simulink library "AerodynamicModel"  (R2024a)
settings: Solver=ode45  StartTime=0.0  StopTime=10.0  RelTol=1e-3  EnableMultiTasking=on
values from neighbouring files (symbols this model uses):
  b = 5.76    [Initialization.m]    (also in Initialization_alt2.m; Initialization_cg1.m; Initialization_loop.m; Initialization_v2.m)
  CD0 = 0.01534    [Initialization.m]    (also in Initialization_alt2.m; Initialization_cg1.m = 0.01532; Initialization_loop.m = 0.01533; Initialization_v2.m)
  CD_alpha = 0    [Initialization.m]    (also in Initialization_alt2.m; Initialization_cg1.m; Initialization_loop.m; Initialization_v2.m)
  CD_elev = 0.000010*180/pi    (= 0.000572957795131)    [Initialization.m]    (also in Initialization_alt2.m; Initialization_cg1.m; Initialization_loop.m; Initialization_v2.m)
  CL0 = 0.20539    [Initialization.m]    (also in Initialization_alt2.m; Initialization_cg1.m; Initialization_loop.m; Initialization_v2.m)
  Cl_ail = 0.005020*180/pi    (= 0.287624813156)    [Initialization.m]    (also in Initialization_alt2.m; Initialization_cg1.m; Initialization_loop.m = 0.276051065694; Initialization_v2.m)
  CL_alpha = 4.865906    [Initialization.m]    (also in Initialization_alt2.m = 4.865879; Initialization_cg1.m; Initialization_loop.m = 4.86588; Initialization_v2.m = 4.865879)
  CL_AlphaDot = 0    [Initialization.m]    (also in Initialization_alt2.m; Initialization_cg1.m; Initialization_loop.m; Initialization_v2.m)
  Cl_beta = -0.020876    [Initialization.m]    (also in Initialization_alt2.m; Initialization_cg1.m; Initialization_loop.m; Initialization_v2.m)
  CL_elev = 0.0064*180/pi    (= 0.366692988884)    [Initialization.m]    (also in Initialization_alt2.m; Initialization_cg1.m; Initialization_loop.m; Initialization_v2.m)
  Cl_p = -0.464911    [Initialization.m]    (also in Initialization_alt2.m; Initialization_cg1.m = -0.464912; Initialization_loop.m; Initialization_v2.m = -0.464912)
  CL_q = 8.057645    [Initialization.m]    (also in Initialization_alt2.m = 7.535819; Initialization_cg1.m = 7.53583; Initialization_loop.m = 8.688618; Initialization_v2.m = 7.535819)
  Cl_r = 0.073227    [Initialization.m]    (also in Initialization_alt2.m = 0.072902; Initialization_cg1.m = 0.099393; Initialization_loop.m = 0.073622; Initialization_v2.m = 0.099393)
  Cl_rud = -0.000235*180/pi    (= -0.0134645081856)    [Initialization.m]    (also in Initialization_alt2.m; Initialization_cg1.m; Initialization_loop.m; Initialization_v2.m)
  Cm0 = -0.05304    [Initialization.m]    (also in Initialization_alt2.m = -0.04206; Initialization_cg1.m = -0.04206; Initialization_loop.m = -0.06631; Initialization_v2.m = -0.04206)
  Cm_alpha = -0.985144    [Initialization.m]    (also in Initialization_alt2.m = -0.724231; Initialization_cg1.m = -0.724233; Initialization_loop.m = -1.300632; Initialization_v2.m = -0.724231)
  Cm_AlphaDot = 0    [Initialization.m]    (also in Initialization_alt2.m; Initialization_cg1.m; Initialization_loop.m; Initialization_v2.m)
  Cm_elev = -0.016898 *180/pi    (= -0.968184082212)    [Initialization.m]    (also in Initialization_alt2.m = -0.948588925619; Initialization_cg1.m = -0.948588925619; Initialization_loop.m = -0.991847239151; Initialization_v2.m = -0.948588925619)
  Cm_q = -9.625909    [Initialization.m]    (also in Initialization_alt2.m = -9.117785; Initialization_cg1.m = -9.117792; Initialization_loop.m = -10.314818; Initialization_v2.m = -9.117785)
  cma = 0.84    [Initialization.m]    (also in Initialization_alt2.m; Initialization_cg1.m; Initialization_loop.m; Initialization_v2.m)
  Cn_ail = 0.000017*180/pi    (= 0.000974028251722)    [Initialization.m]    (also in Initialization_alt2.m = 0.000859436692696; Initialization_cg1.m = 0.000916732472209; Initialization_loop.m = 0.000630253574644; Initialization_v2.m = 0.000859436692696)
  Cn_beta = 0.075240    (= 0.07524)    [Initialization.m]    (also in Initialization_alt2.m = 0.073751; Initialization_cg1.m = 0.073751; Initialization_loop.m = 0.07704; Initialization_v2.m = 0.073751)
  Cn_p = -0.012611    [Initialization.m]    (also in Initialization_alt2.m = -0.012431; Initialization_cg1.m = -0.012466; Initialization_loop.m = -0.012825; Initialization_v2.m = -0.012431)
  Cn_r = -0.076155    [Initialization.m]    (also in Initialization_alt2.m = -0.07368; Initialization_cg1.m = -0.073674; Initialization_loop.m = -0.079209; Initialization_v2.m = -0.07368)
  Cn_rud = 0.001227*180/pi    (= 0.0703019214626)    [Initialization.m]    (also in Initialization_alt2.m = 0.0690414143133; Initialization_cg1.m = 0.0690414143133; Initialization_loop.m = 0.0717916117299; Initialization_v2.m = 0.0690414143133)
  CY_ail = -0.000195*180/pi    (= -0.0111726770051)    [Initialization.m]    (also in Initialization_alt2.m; Initialization_cg1.m; Initialization_loop.m = -0.010828902328; Initialization_v2.m)
  CY_beta = -0.191039    [Initialization.m]    (also in Initialization_alt2.m; Initialization_cg1.m; Initialization_loop.m; Initialization_v2.m)
  CY_p = 0.023084    [Initialization.m]    (also in Initialization_alt2.m; Initialization_cg1.m = 0.023086; Initialization_loop.m; Initialization_v2.m)
  CY_r = 0.170019    [Initialization.m]    (also in Initialization_alt2.m = 0.167041; Initialization_cg1.m = 0.167041; Initialization_loop.m = 0.173621; Initialization_v2.m = 0.167041)
  CY_rud = -0.002799*180/pi    (= -0.160370886857)    [Initialization.m]    (also in Initialization_alt2.m; Initialization_cg1.m; Initialization_loop.m; Initialization_v2.m)
  S = 4.74    [Initialization.m]    (also in Initialization_alt2.m; Initialization_cg1.m; Initialization_loop.m; Initialization_v2.m)
settings Model: Creator=bruno  LastModifiedBy=Marcos Ramalho
settings SolverCC: AlgebraicLoopSolver=TrustRegion
settings DataIOCC: LimitDataPoints=on  ReturnWorkspaceOutputs=off
settings OptimizationCC: LifeSpan=inf
settings DebuggingCC: UnconnectedInputMsg=warning  UnconnectedOutputMsg=warning  UnconnectedLineMsg=warning  AllowSymbolicDim=off  SFUnexpectedBacktrackingDiag=warning  SFNoUnconditionalDefaultTransitionDiag=warning  ArithmeticOperatorsInVariantConditions=warning
settings ModelReferenceCC: EnableRefExpFcnMdlSchedulingChecks=on
settings SFSimCC: SimUseLocalCustomCode=off  CustomCodeUndefinedFunction=UseInterfaceOnly
settings RTWCC: RTWUseLocalCustomCode=off  GPUComputeCapability=3.5
settings CodeAppCC: StateflowObjectComments=on
settings GRTTargetCC: TargetLangStandard=C89/C90 (ANSI)
settings ConfigComp: CovMetricSettings=dw  CovSaveCumulativeToWorkspaceVar=on  CovSaveSingleToWorkspaceVar=on  CovExternalEMLEnable=off

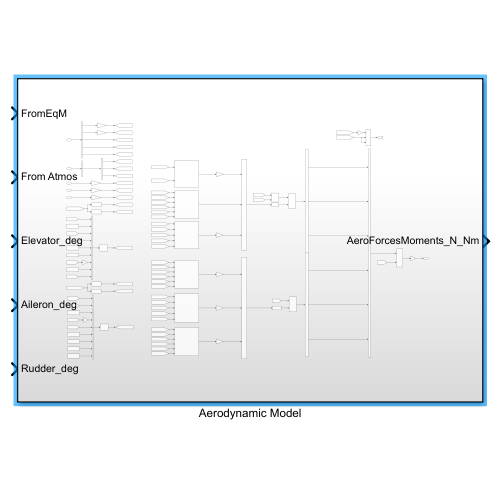
[thumbnail: Simulink's stored preview of the top-level diagram]
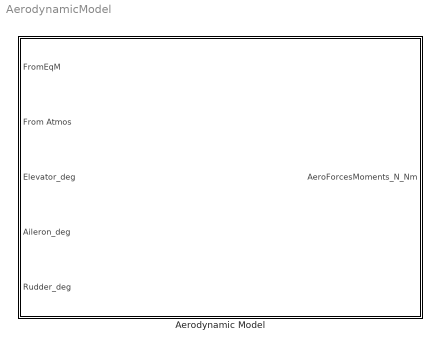
== system AerodynamicModel ==
  Aerodynamic Model : Subsystem

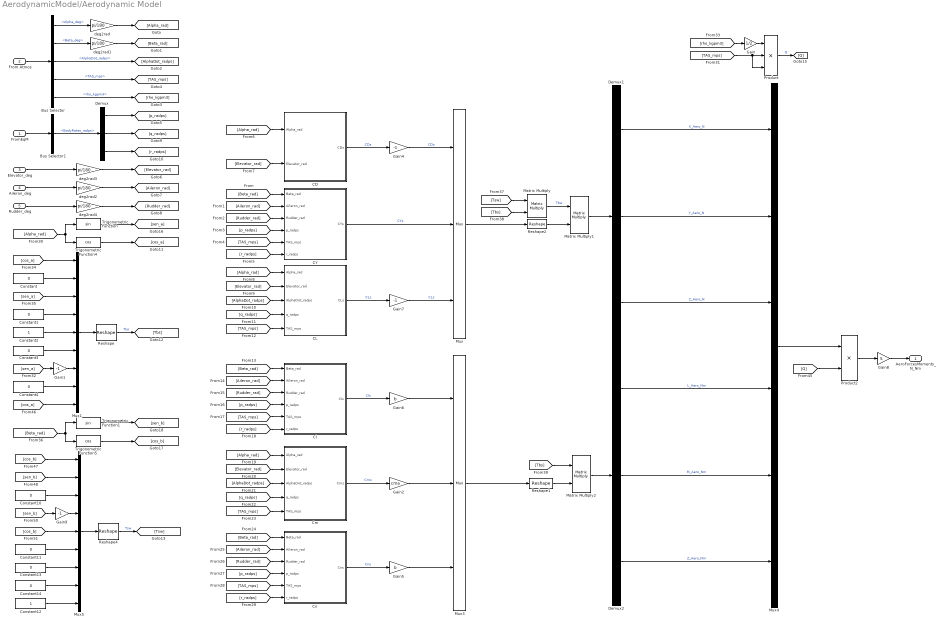
== system AerodynamicModel/Aerodynamic Model ==
  FromEqM : Inport
  From Atmos : Inport  Port=2
  Elevator_deg : Inport  Port=3
  Aileron_deg : Inport  Port=4
  Rudder_deg : Inport  Port=5
  Bus Selector : BusSelector  OutputSignals=Alpha_deg,Beta_deg,AlphaDot_radps,TAS_mps,rho_kgpm3
  Bus Selector1 : BusSelector  OutputSignals=BodyRates_radps
  CD : Subsystem
  CL : Subsystem
  CY : Subsystem
  Cl : Subsystem
  Cm : Subsystem
  Cn : Subsystem
  Constant{,1,3..4,10..11,13..14} (8 alike) : Constant  Value=0
  Constant12 : Constant
  Constant2 : Constant
  Demux : Demux  Outputs=3
  Demux1 : Demux  Outputs=3
  Demux2 : Demux  Outputs=3
  Gain : Gain  Gain=1/2
  Gain{1,4,7,9} (4 alike) : Gain  Gain=-1
  Gain2 : Gain  Gain=cma
  Gain5 : Gain  Gain=b
  Gain6 : Gain  Gain=b
  Gain8 : Gain  Gain=S
  Matrix Multiply : Product  Multiplication=Matrix(*)
  Matrix Multiply1 : Product  Multiplication=Matrix(*)
  Matrix Multiply2 : Product  Multiplication=Matrix(*)
  Mux : Mux  Inputs=3
  Mux1 : Mux  Inputs=9
  Mux3 : Mux  Inputs=3
  Mux4 : Mux  Inputs=6
  Mux5 : Mux  Inputs=9
  Product : Product  Inputs=3
  Product2 : Product
  Reshape : Reshape  OutputDimensionality=Customize  OutputDimensions=[3,3]
  Reshape1 : Reshape  OutputDimensionality=Customize  OutputDimensions=[3,1]
  Reshape2 : Reshape  OutputDimensionality=Customize  OutputDimensions=[3,1]
  Reshape4 : Reshape  OutputDimensionality=Customize  OutputDimensions=[3,3]
  Trigonometric Function : Trigonometry
  Trigonometric Function1 : Trigonometry
  Trigonometric Function4 : Trigonometry  Operator=cos
  Trigonometric Function5 : Trigonometry  Operator=cos
  deg2rad{,1..4} (5 alike) : Gain  Gain=pi/180
  AeroForcesMoments_N_Nm : Outport
  wires:
  Gain9/1 -> Mux5/4
  Constant14/1 -> Mux5/8
  [sen_b] -> Gain9/1
  Constant11/1 -> Mux5/6
  [cos_b] -> Mux5/5
  [sen_b] -> Mux5/2
  Mux5/1 -> Reshape4/1
  Reshape4/1 -> [Tsw]  "Tsw"
  Constant13/1 -> Mux5/7
  Constant10/1 -> Mux5/3
  Constant12/1 -> Mux5/9
  [cos_b] -> Mux5/1
  Trigonometric Function1/1 -> [sen_b]
  [Beta_rad] -> Trigonometric Function1/1, Trigonometric Function5/1
  Trigonometric Function5/1 -> [cos_b]
  Gain8/1 -> AeroForcesMoments_N_Nm/1
  Product2/1 -> Gain8/1
  [Q] -> Product2/2
  Mux4/1 -> Product2/1
  Demux2/3 -> Mux4/6  "Z_Aero_Nm"
  Demux2/2 -> Mux4/5  "M_Aero_Nm"
  Demux2/1 -> Mux4/4  "L_Aero_Nm"
  Demux1/3 -> Mux4/3  "Z_Aero_N"
  Demux1/1 -> Mux4/1  "X_Aero_N"
  Demux1/2 -> Mux4/2  "Y_Aero_N"
  Matrix Multiply2/1 -> Demux2/1
  Matrix Multiply1/1 -> Demux1/1
  [Tbs] -> Matrix Multiply2/1
  Reshape1/1 -> Matrix Multiply2/2
  Mux3/1 -> Reshape1/1
  Gain5/1 -> Mux3/3
  Gain2/1 -> Mux3/2
  Gain6/1 -> Mux3/1
  Gain7/1 -> Mux/3  "CLs"
  Gain4/1 -> Mux/1  "CDs"
  Reshape2/1 -> Matrix Multiply1/2
  Matrix Multiply/1 -> Matrix Multiply1/1  "Tbw"
  [Tbs] -> Matrix Multiply/2
  [Tsw] -> Matrix Multiply/1
  Reshape/1 -> [Tbs]  "Tbs"
  Mux1/1 -> Reshape/1
  [cos_a] -> Mux1/9
  Constant4/1 -> Mux1/8
  Gain1/1 -> Mux1/7
  [sen_a] -> Gain1/1
  Constant3/1 -> Mux1/6
  Constant2/1 -> Mux1/5
  Constant1/1 -> Mux1/4
  [sen_a] -> Mux1/3
  Constant/1 -> Mux1/2
  [cos_a] -> Mux1/1
  Trigonometric Function4/1 -> [cos_a]
  Trigonometric Function/1 -> [sen_a]
  [Alpha_rad] -> Trigonometric Function/1, Trigonometric Function4/1
  Mux/1 -> Reshape2/1
  Bus Selector1/1 -> Demux/1  "<BodyRates_radps>"
  FromEqM/1 -> Bus Selector1/1
  Bus Selector/1 -> deg2rad/1  "<Alpha_deg>"
  From Atmos/1 -> Bus Selector/1
  Demux/3 -> [r_radps]
  deg2rad3/1 -> [Elevator_rad]
  Demux/1 -> [p_radps]
  Demux/2 -> [q_radps]
  Aileron_deg/1 -> deg2rad2/1
  deg2rad2/1 -> [Aileron_rad]
  Bus Selector/2 -> deg2rad1/1  "<Beta_deg>"
  deg2rad4/1 -> [Rudder_rad]
  Elevator_deg/1 -> deg2rad3/1
  Bus Selector/3 -> [AlphaDot_radps]  "<AlphaDot_radps>"
  Rudder_deg/1 -> deg2rad4/1
  deg2rad/1 -> [Alpha_rad]
  deg2rad1/1 -> [Beta_rad]
  Cl/1(Cls) -> Gain6/1  "Cls"
  CD/1(CDs) -> Gain4/1  "CDs"
  [rho_kgpm3] -> Gain/1
  [TAS_mps] -> Product/3, Product/2
  Gain/1 -> Product/1
  CY/1(CYs) -> Mux/2  "CYs"
  Cm/1(Cms) -> Gain2/1  "Cms"
  CL/1(CLs) -> Gain7/1  "CLs"
  Cn/1(Cns) -> Gain5/1  "Cns"
  Product/1 -> [Q]  "Q"
  Bus Selector/4 -> [TAS_mps]  "<TAS_mps>"
  Bus Selector/5 -> [rho_kgpm3]  "<rho_kgpm3>"
  [Beta_rad] -> CY/1(Beta_rad)
  [Aileron_rad] -> CY/2(Aileron_rad)
  [Rudder_rad] -> CY/3(Rudder_rad)
  [p_radps] -> CY/4(p_radps)
  [TAS_mps] -> CY/5(TAS_mps)
  [r_radps] -> CY/6(r_radps)
  [Alpha_rad] -> CD/1(Alpha_rad)
  [Elevator_rad] -> CD/2(Elevator_rad)
  [Alpha_rad] -> CL/1(Alpha_rad)
  [Elevator_rad] -> CL/2(Elevator_rad)
  [AlphaDot_radps] -> CL/3(AlphaDot_radps)
  [q_radps] -> CL/4(q_radps)
  [TAS_mps] -> CL/5(TAS_mps)
  [Beta_rad] -> Cl/1(Beta_rad)
  [Aileron_rad] -> Cl/2(Aileron_rad)
  [Rudder_rad] -> Cl/3(Rudder_rad)
  [p_radps] -> Cl/4(p_radps)
  [TAS_mps] -> Cl/5(TAS_mps)
  [r_radps] -> Cl/6(r_radps)
  [Alpha_rad] -> Cm/1(Alpha_rad)
  [Elevator_rad] -> Cm/2(Elevator_rad)
  [AlphaDot_radps] -> Cm/3(AlphaDot_radps)
  [q_radps] -> Cm/4(q_radps)
  [TAS_mps] -> Cm/5(TAS_mps)
  [Beta_rad] -> Cn/1(Beta_rad)
  [Aileron_rad] -> Cn/2(Aileron_rad)
  [Rudder_rad] -> Cn/3(Rudder_rad)
  [p_radps] -> Cn/4(p_radps)
  [TAS_mps] -> Cn/5(TAS_mps)
  [r_radps] -> Cn/6(r_radps)

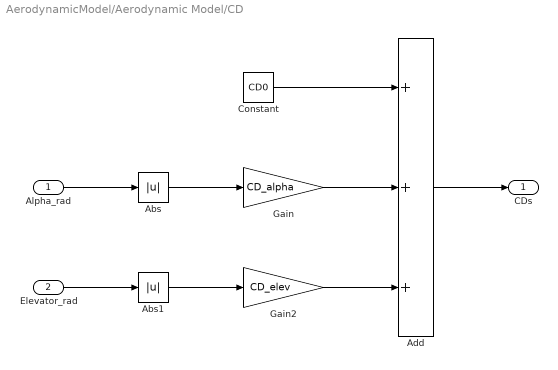
== system AerodynamicModel/Aerodynamic Model/CD ==
  Alpha_rad : Inport
  Elevator_rad : Inport  Port=2
  Abs : Abs  SaturateOnIntegerOverflow=off
  Abs1 : Abs  SaturateOnIntegerOverflow=off
  Add : Sum  Inputs=+++
  Constant : Constant  Value=CD0
  Gain : Gain  Gain=CD_alpha
  Gain2 : Gain  Gain=CD_elev
  CDs : Outport
  wires:
  Gain2/1 -> Add/3
  Abs1/1 -> Gain2/1
  Abs/1 -> Gain/1
  Constant/1 -> Add/1
  Elevator_rad/1 -> Abs1/1
  Add/1 -> CDs/1
  Alpha_rad/1 -> Abs/1
  Gain/1 -> Add/2

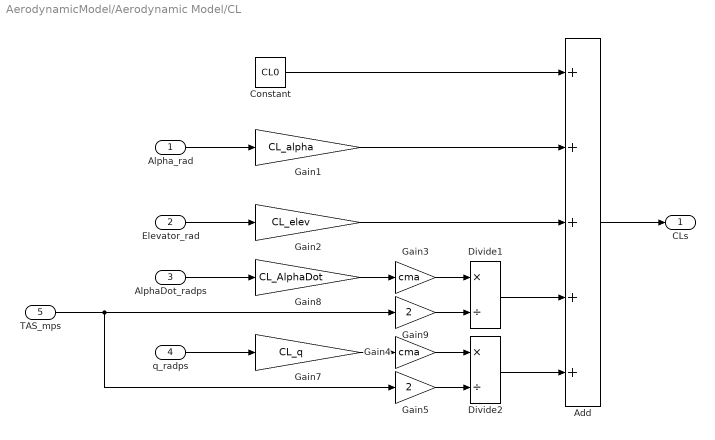
== system AerodynamicModel/Aerodynamic Model/CL ==
  Alpha_rad : Inport
  Elevator_rad : Inport  Port=2
  AlphaDot_radps : Inport  Port=3
  q_radps : Inport  Port=4
  TAS_mps : Inport  Port=5
  Add : Sum  Inputs=+++++
  Constant : Constant  Value=CL0
  Divide1 : Product  Inputs=*/
  Divide2 : Product  Inputs=*/
  Gain1 : Gain  Gain=CL_alpha
  Gain2 : Gain  Gain=CL_elev
  Gain3 : Gain  Gain=cma
  Gain4 : Gain  Gain=cma
  Gain5 : Gain  Gain=2
  Gain7 : Gain  Gain=CL_q
  Gain8 : Gain  Gain=CL_AlphaDot
  Gain9 : Gain  Gain=2
  CLs : Outport
  wires:
  Gain2/1 -> Add/3
  Divide1/1 -> Add/4
  Gain9/1 -> Divide1/2
  Gain3/1 -> Divide1/1
  Gain8/1 -> Gain3/1
  Divide2/1 -> Add/5
  Gain5/1 -> Divide2/2
  TAS_mps/1 -> Gain9/1, Gain5/1
  Gain4/1 -> Divide2/1
  Gain7/1 -> Gain4/1
  Add/1 -> CLs/1
  Alpha_rad/1 -> Gain1/1
  Constant/1 -> Add/1
  Gain1/1 -> Add/2
  q_radps/1 -> Gain7/1
  Elevator_rad/1 -> Gain2/1
  AlphaDot_radps/1 -> Gain8/1

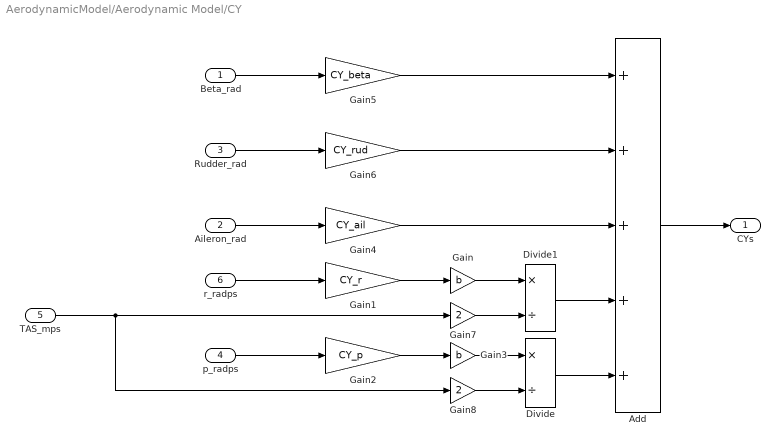
== system AerodynamicModel/Aerodynamic Model/CY ==
  Beta_rad : Inport
  Aileron_rad : Inport  Port=2
  Rudder_rad : Inport  Port=3
  p_radps : Inport  Port=4
  TAS_mps : Inport  Port=5
  r_radps : Inport  Port=6
  Add : Sum  Inputs=+++++
  Divide : Product  Inputs=*/
  Divide1 : Product  Inputs=*/
  Gain : Gain  Gain=b
  Gain1 : Gain  Gain=CY_r
  Gain2 : Gain  Gain=CY_p
  Gain3 : Gain  Gain=b
  Gain4 : Gain  Gain=CY_ail
  Gain5 : Gain  Gain=CY_beta
  Gain6 : Gain  Gain=CY_rud
  Gain7 : Gain  Gain=2
  Gain8 : Gain  Gain=2
  CYs : Outport
  wires:
  Gain4/1 -> Add/3
  Gain6/1 -> Add/2
  r_radps/1 -> Gain1/1
  Rudder_rad/1 -> Gain6/1
  Gain5/1 -> Add/1
  Divide1/1 -> Add/4
  Gain1/1 -> Gain/1
  Gain3/1 -> Divide/1
  Gain8/1 -> Divide/2
  Gain7/1 -> Divide1/2
  Gain/1 -> Divide1/1
  Add/1 -> CYs/1
  Divide/1 -> Add/5
  TAS_mps/1 -> Gain8/1, Gain7/1
  Beta_rad/1 -> Gain5/1
  Gain2/1 -> Gain3/1
  p_radps/1 -> Gain2/1
  Aileron_rad/1 -> Gain4/1

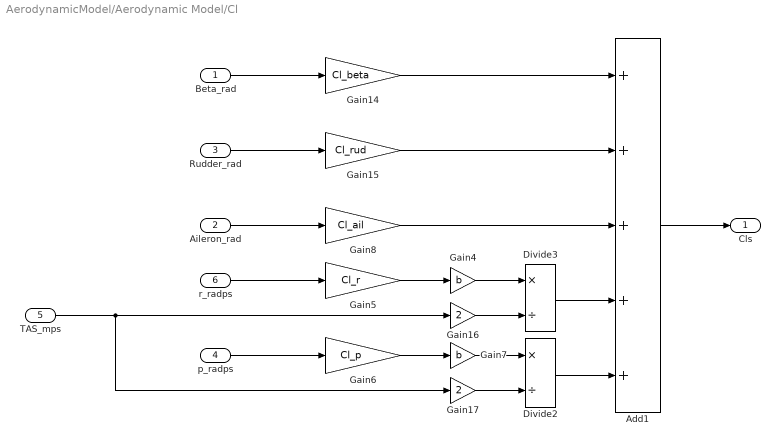
== system AerodynamicModel/Aerodynamic Model/Cl ==
  Beta_rad : Inport
  Aileron_rad : Inport  Port=2
  Rudder_rad : Inport  Port=3
  p_radps : Inport  Port=4
  TAS_mps : Inport  Port=5
  r_radps : Inport  Port=6
  Add1 : Sum  Inputs=+++++
  Divide2 : Product  Inputs=*/
  Divide3 : Product  Inputs=*/
  Gain14 : Gain  Gain=Cl_beta
  Gain15 : Gain  Gain=Cl_rud
  Gain16 : Gain  Gain=2
  Gain17 : Gain  Gain=2
  Gain4 : Gain  Gain=b
  Gain5 : Gain  Gain=Cl_r
  Gain6 : Gain  Gain=Cl_p
  Gain7 : Gain  Gain=b
  Gain8 : Gain  Gain=Cl_ail
  Cls : Outport
  wires:
  Gain8/1 -> Add1/3
  Beta_rad/1 -> Gain14/1
  Gain4/1 -> Divide3/1
  Gain14/1 -> Add1/1
  Gain5/1 -> Gain4/1
  Gain7/1 -> Divide2/1
  Gain15/1 -> Add1/2
  Gain17/1 -> Divide2/2
  Gain16/1 -> Divide3/2
  Aileron_rad/1 -> Gain8/1
  TAS_mps/1 -> Gain17/1, Gain16/1
  Divide2/1 -> Add1/5
  Gain6/1 -> Gain7/1
  r_radps/1 -> Gain5/1
  Rudder_rad/1 -> Gain15/1
  Divide3/1 -> Add1/4
  p_radps/1 -> Gain6/1
  Add1/1 -> Cls/1

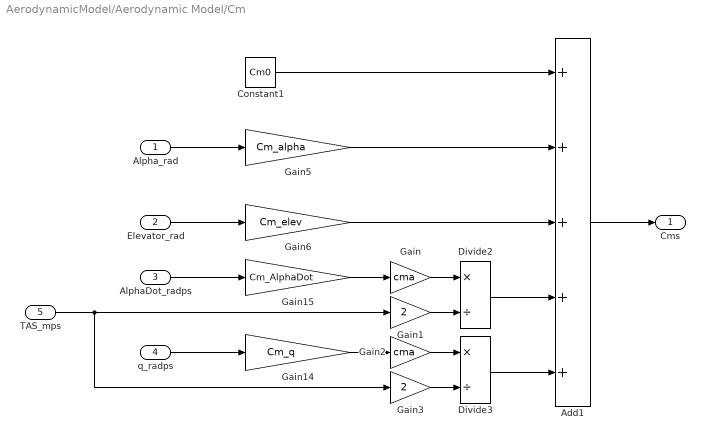
== system AerodynamicModel/Aerodynamic Model/Cm ==
  Alpha_rad : Inport
  Elevator_rad : Inport  Port=2
  AlphaDot_radps : Inport  Port=3
  q_radps : Inport  Port=4
  TAS_mps : Inport  Port=5
  Add1 : Sum  Inputs=+++++
  Constant1 : Constant  Value=Cm0
  Divide2 : Product  Inputs=*/
  Divide3 : Product  Inputs=*/
  Gain : Gain  Gain=cma
  Gain1 : Gain  Gain=2
  Gain14 : Gain  Gain=Cm_q
  Gain15 : Gain  Gain=Cm_AlphaDot
  Gain2 : Gain  Gain=cma
  Gain3 : Gain  Gain=2
  Gain5 : Gain  Gain=Cm_alpha
  Gain6 : Gain  Gain=Cm_elev
  Cms : Outport
  wires:
  Gain6/1 -> Add1/3
  Gain14/1 -> Gain2/1
  AlphaDot_radps/1 -> Gain15/1
  Gain3/1 -> Divide3/2
  Gain2/1 -> Divide3/1
  Divide3/1 -> Add1/5
  Constant1/1 -> Add1/1
  Divide2/1 -> Add1/4
  TAS_mps/1 -> Gain1/1, Gain3/1
  Elevator_rad/1 -> Gain6/1
  Gain1/1 -> Divide2/2
  Gain15/1 -> Gain/1
  Gain5/1 -> Add1/2
  Add1/1 -> Cms/1
  Alpha_rad/1 -> Gain5/1
  Gain/1 -> Divide2/1
  q_radps/1 -> Gain14/1

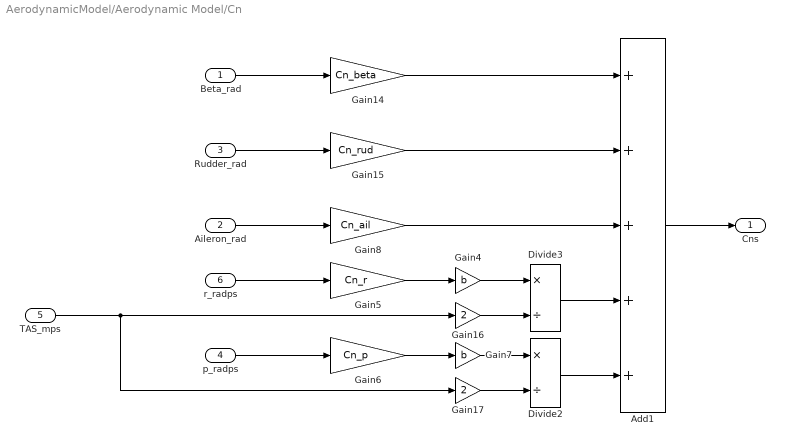
== system AerodynamicModel/Aerodynamic Model/Cn ==
  Beta_rad : Inport
  Aileron_rad : Inport  Port=2
  Rudder_rad : Inport  Port=3
  p_radps : Inport  Port=4
  TAS_mps : Inport  Port=5
  r_radps : Inport  Port=6
  Add1 : Sum  Inputs=+++++
  Divide2 : Product  Inputs=*/
  Divide3 : Product  Inputs=*/
  Gain14 : Gain  Gain=Cn_beta
  Gain15 : Gain  Gain=Cn_rud
  Gain16 : Gain  Gain=2
  Gain17 : Gain  Gain=2
  Gain4 : Gain  Gain=b
  Gain5 : Gain  Gain=Cn_r
  Gain6 : Gain  Gain=Cn_p
  Gain7 : Gain  Gain=b
  Gain8 : Gain  Gain=Cn_ail
  Cns : Outport
  wires:
  Gain15/1 -> Add1/2
  Gain8/1 -> Add1/3
  TAS_mps/1 -> Gain17/1, Gain16/1
  Rudder_rad/1 -> Gain15/1
  Aileron_rad/1 -> Gain8/1
  Divide2/1 -> Add1/5
  Gain4/1 -> Divide3/1
  Gain7/1 -> Divide2/1
  p_radps/1 -> Gain6/1
  Beta_rad/1 -> Gain14/1
  Gain6/1 -> Gain7/1
  Divide3/1 -> Add1/4
  Add1/1 -> Cns/1
  Gain5/1 -> Gain4/1
  r_radps/1 -> Gain5/1
  Gain16/1 -> Divide3/2
  Gain17/1 -> Divide2/2
  Gain14/1 -> Add1/1
